simulink model "transmit_filters_TL"  (R2021a)
settings: Solver=VariableStepAuto  StartTime=0.0  StopTime=0.5  RelTol=1e-3
libraries: commdigbbndpm3 x1, commfilt2 x1, commrandsrc3 x1, dspsigops x1
settings Model: Creator=Tomas  LastModifiedBy=Tomas

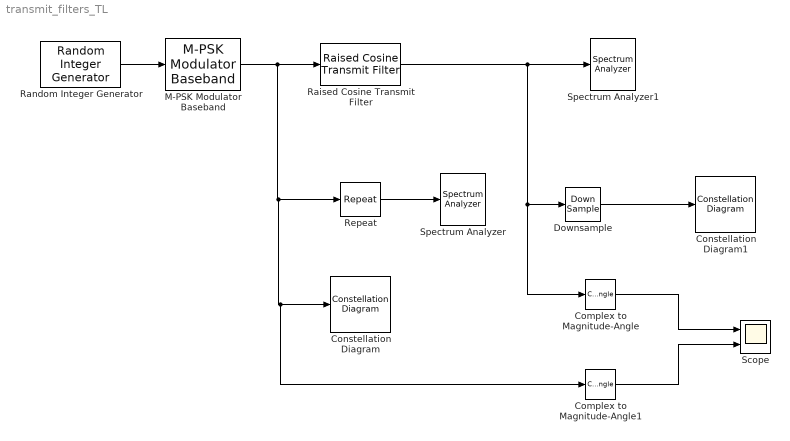
== system transmit_filters_TL ==
  Complex to Magnitude-Angle : ComplexToMagnitudeAngle  Output=Magnitude
  Complex to Magnitude-Angle1 : ComplexToMagnitudeAngle  Output=Magnitude
  Constellation Diagram : ConstellationDiagram
  Constellation Diagram1 : ConstellationDiagram
  Downsample : DownSample  N=8
  M-PSK Modulator Baseband : commdigbbndpm3/M-PSK Modulator Baseband  M=8  InType=Integer  Enc=Gray  Mapping=[0:7]  Ph=pi/8  outDtype=double  outWordLen=16  outUDDataType=sfix(16)  outFracLenMode=Best precision  outFracLen=15  outDataTypeStr=double  outLastDataTypeStr=double
  Raised Cosine Transmit Filter : commfilt2/Raised Cosine Transmit Filter  filtType=Square root  R=0.35  filtSpan=10  N=8  filterGain=1  RateOptions=Allow multirate processing  framing=Mute  checkCoeff=off  variableName=rcTxFilt  checkGain=Normalized  sampMode=Mute  saveAsFlag=0  currentFiltSpan=10  D=(10)/2  launchFVT=on  roundingMode=Floor  overflowMode=off  coeffDataTypeStr=Inherit: Same word length as input  coeffMin=[]  coeffMax=[]  coeffLastDataTypeStr=Inherit: Same word length as input  outputDataTypeStr=Inherit: Same as accumulator  outputMin=[]  outputMax=[]  outputLastDataTypeStr=Inherit: Same as accumulator
  Random Integer Generator : commrandsrc3/Random Integer Generator  SetSize=8  SeedSource=Auto  Seed=0  SampleTime=1/100e3  SamplesPerFrame=1  OutputDataType=double  SimulateUsing=Interpreted execution
  Repeat : dspsigops/Repeat  N=8  InputProcessing=Columns as channels (frame based)  RateOptions=Enforce single-rate processing  ic=0  mode=Unused parameter value
  Scope : Scope  NumInputPorts=2
  Spectrum Analyzer : SpectrumAnalyzer
  Spectrum Analyzer1 : SpectrumAnalyzer
  wires:
  Random Integer Generator/1 -> M-PSK Modulator Baseband/1
  M-PSK Modulator Baseband/1 -> Complex to Magnitude-Angle1/1, Constellation Diagram/1, Repeat/1, Raised Cosine Transmit Filter/1
  Repeat/1 -> Spectrum Analyzer/1
  Raised Cosine Transmit Filter/1 -> Complex to Magnitude-Angle/1, Downsample/1, Spectrum Analyzer1/1
  Downsample/1 -> Constellation Diagram1/1
  Complex to Magnitude-Angle1/1 -> Scope/2
  Complex to Magnitude-Angle/1 -> Scope/1
